simulink model "s_maglev_piv"  (Simulink 7.7)
settings: Solver=ode4  StartTime=0.0  StopTime=10  FixedStep=0.002  RelTol=1e-3
values from neighbouring files (symbols this model uses):
  g = 9.81    [config_maglev.m]
  IC_MAX = 3    [config_maglev.m]
  Kff_b = ic0 / xb0    [d_maglev_pi_piv.m]    (also in setup_maglev.m = 0)
  Ki_b = -p0*wn_b^2*ic0/(2*g)    [d_maglev_pi_piv.m]    (also in setup_maglev.m = 0)
  Ki_c = wn_c^2 * tau_c / Kc_dc    [d_maglev_pi_piv.m]    (also in setup_maglev.m = 0)
  Km = 6.5308e-5    (= 6.5308e-05)    [config_maglev.m]
  Kp_b = -(2*p0*zeta_b*wn_b*xb0 + wn_b^2*xb0+2*g)*ic0/(2*xb0*g)    [d_maglev_pi_piv.m]    (also in setup_maglev.m = 0)
  Kp_c = (2*zeta_c*wn_c*tau_c - 1) / Kc_dc    [d_maglev_pi_piv.m]    (also in setup_maglev.m = 0)
  Kv_b = -(p0+2*zeta_b*wn_b)*ic0/(2*g)    [d_maglev_pi_piv.m]    (also in setup_maglev.m = 0)
  Lc = 0.4125    [config_maglev.m]
  MAX_XB_WDUP = 1    [setup_maglev.m]
  Mb = 0.068    [config_maglev.m]
  Rc = 10    [config_maglev.m]
  Rs = 1    [config_maglev.m]
  Tb = 0.014    [config_maglev.m]
  VMAX_AMP = 24    [config_maglev.m]
  xb0 = 6e-3    (= 0.006)    [setup_maglev.m]
  XB_REF_RATE = 5e-3    (= 0.005)    [setup_maglev.m]
libraries: simulink x1
settings Model: Creator=MLevis  LastModifiedBy=MLevis  ExtModeTrigDuration=5000
settings SolverCC: PositivePriorityOrder=on
settings RTWCC: SystemTargetFile=quarc_win64.tlc  TemplateMakefile=quarc_default_tmf  Description=QUARC Win64 Target  ProcessScript=quarc_win64_make_rtw_hook
settings STFCustomTargetCC: TargetPreCompLibLocation=C:\PROGRA~3\QUARC\lib\2011a\win64\release  FunctionExecutionProfile=off  GeneratePreprocessorConditionals=Disable all  SystemTargetFile=quarc_win64.tlc
settings GRTTargetCC: TargetPreCompLibLocation=C:\PROGRA~3\QUARC\lib\2011a\win64\release  ParMdlRefBuildCompliant=off  CompOptLevelCompliant=off  MatFileLogging=off  ExtMode=on  ExtModeMexFile=quarc_comm

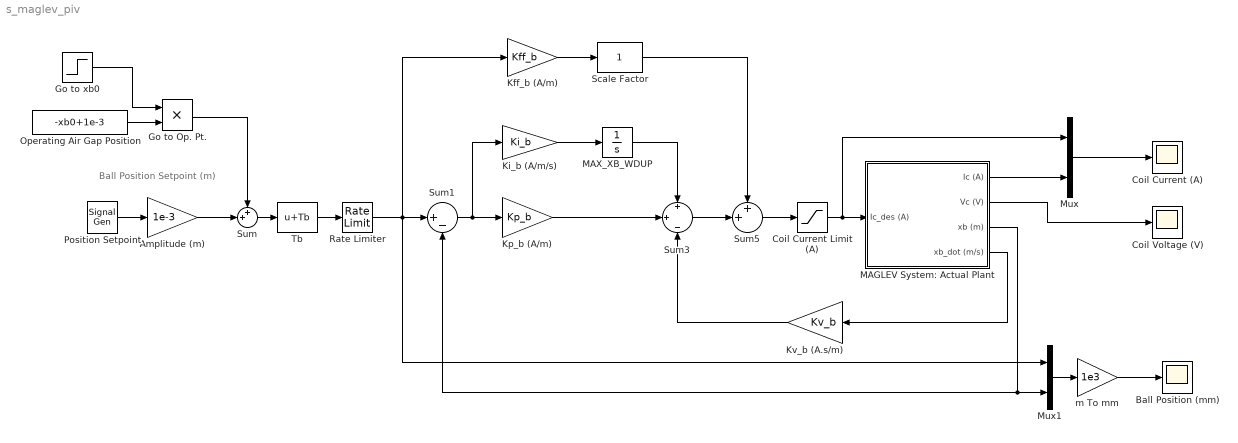
== system s_maglev_piv ==
  note: Ball Position Setpoint (m)
  Amplitude (m) : Gain  Gain=1e-3  SaturateOnIntegerOverflow=on  OutDataTypeStr=Inherit: Same as input  ParamDataTypeStr=Inherit: Same as input
  Ball Position (mm) : Scope
      settings: TimeRange=10  YMin=5  YMax=15  SaveName=data_xb  DataFormat=Array
  Coil Current Limit (A) : Saturate  UpperLimit=IC_MAX  LowerLimit=0
  Coil Current (A) : Scope
      settings: TimeRange=10  YMin=0  YMax=3  SaveName=data_Ic  DataFormat=Array
  Coil Voltage (V) : Scope
      settings: TimeRange=10  YMin=5  YMax=25  SaveName=data_Vc  DataFormat=Array
  Go to Op. Pt. : Product  RndMeth=Zero
  Go to xb0 : Step  Time=2  SampleTime=0
  Kff_b (A/m) : Gain  Gain=Kff_b  SaturateOnIntegerOverflow=on  OutDataTypeStr=Inherit: Same as input  ParamDataTypeStr=Inherit: Same as input
  Ki_b (A/m/s) : Gain  Gain=Ki_b  SaturateOnIntegerOverflow=on  OutDataTypeStr=Inherit: Same as input  ParamDataTypeStr=Inherit: Same as input
  Kp_b (A/m) : Gain  Gain=Kp_b  SaturateOnIntegerOverflow=on  OutDataTypeStr=Inherit: Same as input  ParamDataTypeStr=Inherit: Same as input
  Kv_b (A.s/m) : Gain  Gain=Kv_b  SaturateOnIntegerOverflow=on  OutDataTypeStr=Inherit: Same as input  ParamDataTypeStr=Inherit: Same as input
  MAGLEV System: Actual Plant : Subsystem
  MAX_XB_WDUP : Integrator  LimitOutput=on  UpperSaturationLimit=MAX_XB_WDUP  LowerSaturationLimit=-MAX_XB_WDUP
  Mux : Mux  Inputs=2
  Mux1 : Mux  Inputs=2
  Operating Air Gap Position : Constant  Value=-xb0+1e-3
  Position Setpoint : SignalGenerator  WaveForm=square  Frequency=.25
  Rate Limiter : RateLimiter  RisingSlewLimit=XB_REF_RATE  FallingSlewLimit=-XB_REF_RATE  SampleTimeMode=inherited
  Scale Factor : simulink/Math Operations/Slider Gain  SystemSampleTime=-1  low=0  gain=1  high=1
  Sum : Sum  Inputs=++|
  Sum1 : Sum  Inputs=|+-  SaturateOnIntegerOverflow=on  InputSameDT=on  OutDataTypeStr=Inherit: Same as first input
  Sum3 : Sum  Inputs=+|+|-  SaturateOnIntegerOverflow=on  InputSameDT=on  OutDataTypeStr=Inherit: Same as first input
  Sum5 : Sum  Inputs=++|  SaturateOnIntegerOverflow=on  InputSameDT=on  OutDataTypeStr=Inherit: Same as first input
  Tb : Bias  Bias=Tb
  m To mm : Gain  Gain=1e3  SaturateOnIntegerOverflow=on  OutDataTypeStr=Inherit: Same as input  ParamDataTypeStr=Inherit: Same as input
  wires:
  Sum1/1 -> Ki_b (A/m/s)/1, Kp_b (A/m)/1
  Mux1/1 -> m To mm/1
  Ki_b (A/m/s)/1 -> MAX_XB_WDUP/1
  MAX_XB_WDUP/1 -> Sum3/1
  Kp_b (A/m)/1 -> Sum3/2
  Sum3/1 -> Sum5/2
  Kv_b (A.s/m)/1 -> Sum3/3
  Kff_b (A/m)/1 -> Scale Factor/1
  Mux/1 -> Coil Current (A)/1
  MAGLEV System: Actual Plant/1(Ic (A)) -> Mux/2
  MAGLEV System: Actual Plant/4(xb_dot (m/s)) -> Kv_b (A.s/m)/1
  MAGLEV System: Actual Plant/3(xb (m)) -> Mux1/2, Sum1/2
  Position Setpoint/1 -> Amplitude (m)/1
  Coil Current Limit (A)/1 -> MAGLEV System: Actual Plant/1(Ic_des (A)), Mux/1
  m To mm/1 -> Ball Position (mm)/1
  Sum5/1 -> Coil Current Limit (A)/1
  MAGLEV System: Actual Plant/2(Vc (V)) -> Coil Voltage (V)/1
  Scale Factor/1 -> Sum5/1
  Operating Air Gap Position/1 -> Go to Op. Pt./2
  Sum/1 -> Tb/1
  Tb/1 -> Rate Limiter/1
  Go to xb0/1 -> Go to Op. Pt./1
  Amplitude (m)/1 -> Sum/2
  Go to Op. Pt./1 -> Sum/1
  Rate Limiter/1 -> Sum1/1, Kff_b (A/m)/1, Mux1/1

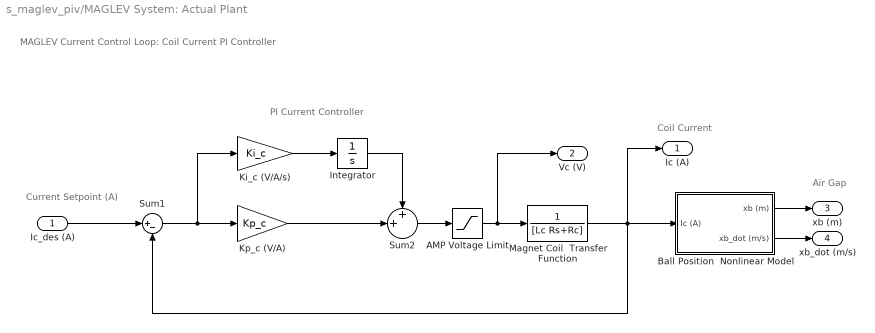
== system s_maglev_piv/MAGLEV System: Actual Plant ==
  note: Coil Current
  note: Air Gap
  note: MAGLEV Current Control Loop:
      | Coil Current PI Controller
  note: Current Setpoint (A)
  note: PI Current Controller
  Ic_des (A) : Inport
  AMP Voltage Limit : Saturate  UpperLimit=VMAX_AMP  LowerLimit=-VMAX_AMP
  Ball Position  Nonlinear Model : Subsystem
  Integrator : Integrator  LimitOutput=on  UpperSaturationLimit=VMAX_AMP  LowerSaturationLimit=-VMAX_AMP
  Ki_c (V/A/s) : Gain  Gain=Ki_c  SaturateOnIntegerOverflow=on  OutDataTypeStr=Inherit: Same as input  ParamDataTypeStr=Inherit: Same as input
  Kp_c (V/A) : Gain  Gain=Kp_c  SaturateOnIntegerOverflow=on  OutDataTypeStr=Inherit: Same as input  ParamDataTypeStr=Inherit: Same as input
  Magnet Coil  Transfer Function : TransferFcn  Denominator=[Lc Rs+Rc]
  Sum1 : Sum  Inputs=|+-
  Sum2 : Sum  Inputs=++|  SaturateOnIntegerOverflow=on  InputSameDT=on  OutDataTypeStr=Inherit: Same as first input
  Ic (A) : Outport  InitialOutput=0
  Vc (V) : Outport  Port=2  InitialOutput=0
  xb (m) : Outport  Port=3  InitialOutput=0
  xb_dot (m/s) : Outport  Port=4  InitialOutput=0
  wires:
  AMP Voltage Limit/1 -> Magnet Coil  Transfer Function/1, Vc (V)/1
  Ki_c (V/A/s)/1 -> Integrator/1
  Integrator/1 -> Sum2/1
  Sum2/1 -> AMP Voltage Limit/1
  Kp_c (V/A)/1 -> Sum2/2
  Ball Position  Nonlinear Model/1(xb (m)) -> xb (m)/1
  Ball Position  Nonlinear Model/2(xb_dot (m/s)) -> xb_dot (m/s)/1
  Magnet Coil  Transfer Function/1 -> Ball Position  Nonlinear Model/1(Ic (A)), Ic (A)/1, Sum1/2
  Sum1/1 -> Ki_c (V/A/s)/1, Kp_c (V/A)/1
  Ic_des (A)/1 -> Sum1/1

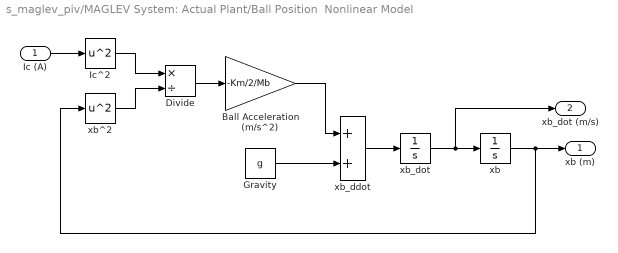
== system s_maglev_piv/MAGLEV System: Actual Plant/Ball Position  Nonlinear Model ==
  Ic (A) : Inport
  Ball Acceleration (m/s^2) : Gain  Gain=-Km/2/Mb
  Divide : Product  Inputs=*/
  Gravity : Constant  Value=g
  Ic^2 : Math  Operator=square  SaturateOnIntegerOverflow=on
  xb : Integrator  InitialCondition=Tb  LimitOutput=on  UpperSaturationLimit=Tb  LowerSaturationLimit=0
  xb^2 : Math  Operator=square  SaturateOnIntegerOverflow=on
  xb_ddot : Sum
  xb_dot : Integrator
  xb (m) : Outport
  xb_dot (m/s) : Outport  Port=2
  wires:
  xb^2/1 -> Divide/2
  Ic (A)/1 -> Ic^2/1
  Divide/1 -> Ball Acceleration (m/s^2)/1
  Ic^2/1 -> Divide/1
  Ball Acceleration (m/s^2)/1 -> xb_ddot/1
  Gravity/1 -> xb_ddot/2
  xb_ddot/1 -> xb_dot/1
  xb_dot/1 -> xb/1, xb_dot (m/s)/1
  xb/1 -> xb (m)/1, xb^2/1
